simulink subsystem "Controls"  (R2024b)
settings: Solver=VariableStepAuto  StartTime=0.0  StopTime=10.0  RelTol=1e-3
undefined symbols (not defined in the file): D1, DiscIntNeverNeededParam, lag, Tctrl, test_alpha, Ts, Yg
libraries: powerlib_extras x74, simulink x10
(part 7 of 7)

== system Controls/Pole 2 Rectifier Control and Protection/Rectifier Controller/Voltage Regulator/Voltage Regulator/Kp Linearisation ==
  note: Kp Linearization
  Alpha_lin : Inport
  Kp : Inport  Port=2
  Inv : Inport  Port=3
  Min_lin : Inport  Port=4
  Max_lin : Inport  Port=5
  Constant3 : Constant  Value=On_lin
  Data Type Conversion : DataTypeConversion  OutDataTypeStr=boolean
  Logical Operator : Logic  Operator=NOT
  Logical Operator1 : Logic  Operator=NOT
  Math Function : Math  Operator=reciprocal  SignedPower=on
  Prod2 : Product  Inputs=3  InputSameDT=on  SaturateOnIntegerOverflow=on  OutDataTypeStr=Inherit: Same as first input
  S6 : Subsystem  mask(Limiter with External Limits){}
      mask Display: disp('      Limiter\n')
  Switch : Switch  Threshold=0.5
  Switch1 : Switch  Threshold=0.5
  Trigonometric Function : Trigonometry
  Trigonometric Function1 : Trigonometry
  k : Gain  Gain=pi/180  SaturateOnIntegerOverflow=on  OutDataTypeStr=Inherit: Same as input  ParamDataTypeStr=Inherit: Same as input
  k1 : Gain  Gain=pi/180  SaturateOnIntegerOverflow=on  OutDataTypeStr=Inherit: Same as input  ParamDataTypeStr=Inherit: Same as input
  Kp_lin : Outport  InitialOutput=0
  wires:
  Min_lin/1 -> S6/3(MIN), Switch/1
  Max_lin/1 -> S6/1(MAX), Switch/3
  Alpha_lin/1 -> S6/2(In)
  Math Function/1 -> Prod2/2
  Trigonometric Function1/1 -> Math Function/1
  k/1 -> Trigonometric Function1/1
  Kp/1 -> Prod2/3, Switch1/1
  Inv/1 -> Logical Operator/1
  Logical Operator/1 -> Switch/2
  Trigonometric Function/1 -> Prod2/1
  S6/1("  ") -> k/1
  k1/1 -> Trigonometric Function/1
  Switch/1 -> k1/1
  Switch1/1 -> Kp_lin/1
  Prod2/1 -> Switch1/3
  Logical Operator1/1 -> Switch1/2  "Off"
  Constant3/1 -> Data Type Conversion/1
  Data Type Conversion/1 -> Logical Operator1/1

== system Controls/Pole 2 Rectifier Control and Protection/Rectifier Controller/Voltage Regulator/Voltage Regulator/S16 ==
  note: INTEGRATOR with External limits & Reset & Hold
  note: Gain * dt
  Max : Inport
  Min : Inport  Port=2
  In : Inport  Port=3
  Reset : Inport  Port=4
  Hold : Inport  Port=5
  Reset Value : Inport  Port=6
  Gain1 : Gain  Gain=k*st  SaturateOnIntegerOverflow=on  OutDataTypeStr=Inherit: Same as input  ParamDataTypeStr=Inherit: Same as input
  IC = ic : UnitDelay  InitialCondition=ic  SampleTime=st  HasFrameUpgradeWarning=on
  Logical Operator4 : Logic  Operator=OR
  MinMax : MinMax  Inputs=2  InputSameDT=on  SaturateOnIntegerOverflow=on
  MinMax1 : MinMax  Function=max  Inputs=2  InputSameDT=on  SaturateOnIntegerOverflow=on
  S6 : Subsystem  mask(Limiter with External Limits){}
      mask Display: disp('      Limiter\n')
  Sum : Sum  InputSameDT=on  SaturateOnIntegerOverflow=on  OutDataTypeStr=Inherit: Same as first input
  Switch2 : Switch  Threshold=0.5
  Switch3 : Switch  Threshold=0.5
  Switch7 : Switch  Threshold=0.5
  Out : Outport  InitialOutput=0
  wires:
  Gain1/1 -> Sum/1
  In/1 -> Gain1/1
  Sum/1 -> S6/2(In)
  S6/1("  ") -> Out/1, IC = ic/1
  Hold/1 -> Logical Operator4/1
  Reset/1 -> Switch7/2, Logical Operator4/2
  Logical Operator4/1 -> Switch2/2, Switch3/2
  Switch2/1 -> MinMax/1
  Max/1 -> Switch2/3, MinMax/2
  Reset Value/1 -> Switch7/1
  MinMax/1 -> S6/1(MAX)
  MinMax1/1 -> S6/3(MIN)
  Switch3/1 -> MinMax1/1
  Min/1 -> Switch3/3, MinMax1/2
  IC = ic/1 -> Switch7/3
  Switch7/1 -> Switch2/1, Sum/2, Switch3/1

== system Controls/Pole 2 Rectifier Control and Protection/Rectifier Controller/Voltage Regulator/Voltage Regulator/S6 ==
  note: Limiter
      | with external
      | limits
  MAX : Inport
  In : Inport  Port=2
  MIN : Inport  Port=3
  MinMax : MinMax  Function=max  Inputs=2  InputSameDT=on  SaturateOnIntegerOverflow=on
  MinMax1 : MinMax  Inputs=2  InputSameDT=on  SaturateOnIntegerOverflow=on
  "  " : Outport  InitialOutput=0
  wires:
  In/1 -> MinMax1/2
  MinMax/1 -> "  "/1
  MIN/1 -> MinMax/1
  MAX/1 -> MinMax1/1
  MinMax1/1 -> MinMax/2

== system Controls/Pole 2 Rectifier Control and Protection/Rectifier Protections/DC Fault Protection (DCPROT)/Enabled Subsystem/Discrete Off Delay ==
  note: Discrete On/Off Delay
  note: Silvano Casoria
      | Power System Simulation Laboratory
      | IREQ, Hydro-Quebc
  IN : Inport
  Constant : Constant
  Constant1 : Constant  Value=delay - eps
  Constant2 : Constant  Value=type_delay
  Data Type Conversion1 : DataTypeConversion  OutDataTypeStr=boolean
  Logical Operator1 : Logic  Operator=OR
  Logical Operator2 : Logic  Operator=NOT  Inputs=1
  OFF Delay : Subsystem  TreatAsAtomicUnit=on
  ON Delay : Subsystem  TreatAsAtomicUnit=on
  Relational Operator1 : RelationalOperator  Operator===
  OUT : Outport  VectorParamsAs1DForOutWhenUnconnected=off
  wires:
  IN/1 -> Data Type Conversion1/1
  Constant1/1 -> OFF Delay/2(DELAY), ON Delay/2(DELAY)
  Logical Operator1/1 -> OUT/1
  ON Delay/1(OUT) -> Logical Operator1/1
  OFF Delay/1(OUT) -> Logical Operator1/2
  Logical Operator2/1 -> ?
  Constant2/1 -> Relational Operator1/1
  Relational Operator1/1 -> Logical Operator2/1, ON Delay/Enable
  Constant/1 -> Relational Operator1/2
  Data Type Conversion1/1 -> OFF Delay/1(IN), ON Delay/1(IN)

== system Controls/Pole 1 Inverter Control and Protection/Inverter Current //Voltage//Gamma Controller /Gamma Regulator/Gamma Regulator/Kp Linearisation/S6 ==
  note: Limiter
      | with external
      | limits
  MAX : Inport
  In : Inport  Port=2
  MIN : Inport  Port=3
  MinMax : MinMax  Function=max  Inputs=2  InputSameDT=on  SaturateOnIntegerOverflow=on
  MinMax1 : MinMax  Inputs=2  InputSameDT=on  SaturateOnIntegerOverflow=on
  "  " : Outport  InitialOutput=0
  wires:
  MinMax1/1 -> MinMax/2
  MAX/1 -> MinMax1/1
  MIN/1 -> MinMax/1
  MinMax/1 -> "  "/1
  In/1 -> MinMax1/2

== system Controls/Pole 1 Inverter Control and Protection/Inverter Current //Voltage//Gamma Controller /Gamma Regulator/Gamma Regulator/S16/S6 ==
  note: Silvano Casoria
      | Laboratoire simulation de reseaux, IREQ
  note: Limiter
      | with external
      | limits
  MAX : Inport
  In : Inport  Port=2
  MIN : Inport  Port=3
  MinMax : MinMax  Function=max  Inputs=2  InputSameDT=on  SaturateOnIntegerOverflow=on
  MinMax1 : MinMax  Inputs=2  InputSameDT=on  SaturateOnIntegerOverflow=on
  "  " : Outport  InitialOutput=0
  wires:
  In/1 -> MinMax1/2
  MinMax/1 -> "  "/1
  MIN/1 -> MinMax/1
  MAX/1 -> MinMax1/1
  MinMax1/1 -> MinMax/2

== system Controls/Pole 1 Inverter Control and Protection/Inverter Current //Voltage//Gamma Controller /Voltage Regulator/Voltage Regulator/Kp Linearisation/S6 ==
  note: Limiter
      | with external
      | limits
  MAX : Inport
  In : Inport  Port=2
  MIN : Inport  Port=3
  MinMax : MinMax  Function=max  Inputs=2  InputSameDT=on  SaturateOnIntegerOverflow=on
  MinMax1 : MinMax  Inputs=2  InputSameDT=on  SaturateOnIntegerOverflow=on
  "  " : Outport  InitialOutput=0
  wires:
  In/1 -> MinMax1/2
  MinMax/1 -> "  "/1
  MIN/1 -> MinMax/1
  MAX/1 -> MinMax1/1
  MinMax1/1 -> MinMax/2

== system Controls/Pole 1 Inverter Control and Protection/Inverter Current //Voltage//Gamma Controller /Voltage Regulator/Voltage Regulator/S16/S6 ==
  note: Limiter
      | with external
      | limits
  note: Silvano Casoria
      | Laboratoire simulation de reseaux, IREQ
  MAX : Inport
  In : Inport  Port=2
  MIN : Inport  Port=3
  MinMax : MinMax  Function=max  Inputs=2  InputSameDT=on  SaturateOnIntegerOverflow=on
  MinMax1 : MinMax  Inputs=2  InputSameDT=on  SaturateOnIntegerOverflow=on
  "  " : Outport  InitialOutput=0
  wires:
  MinMax1/1 -> MinMax/2
  MAX/1 -> MinMax1/1
  MIN/1 -> MinMax/1
  MinMax/1 -> "  "/1
  In/1 -> MinMax1/2

== system Controls/Pole 1 Rectifier Control and Protection/Rectifier Controller/Gamma Regulator/Gamma Regulator/Kp Linearisation/S6 ==
  note: Limiter
      | with external
      | limits
  MAX : Inport
  In : Inport  Port=2
  MIN : Inport  Port=3
  MinMax : MinMax  Function=max  Inputs=2  InputSameDT=on  SaturateOnIntegerOverflow=on
  MinMax1 : MinMax  Inputs=2  InputSameDT=on  SaturateOnIntegerOverflow=on
  "  " : Outport  InitialOutput=0
  wires:
  MinMax1/1 -> MinMax/2
  MAX/1 -> MinMax1/1
  MIN/1 -> MinMax/1
  MinMax/1 -> "  "/1
  In/1 -> MinMax1/2

== system Controls/Pole 1 Rectifier Control and Protection/Rectifier Controller/Gamma Regulator/Gamma Regulator/S16/S6 ==
  note: Silvano Casoria
      | Laboratoire simulation de reseaux, IREQ
  note: Limiter
      | with external
      | limits
  MAX : Inport
  In : Inport  Port=2
  MIN : Inport  Port=3
  MinMax : MinMax  Function=max  Inputs=2  InputSameDT=on  SaturateOnIntegerOverflow=on
  MinMax1 : MinMax  Inputs=2  InputSameDT=on  SaturateOnIntegerOverflow=on
  "  " : Outport  InitialOutput=0
  wires:
  In/1 -> MinMax1/2
  MinMax/1 -> "  "/1
  MIN/1 -> MinMax/1
  MAX/1 -> MinMax1/1
  MinMax1/1 -> MinMax/2

== system Controls/Pole 1 Rectifier Control and Protection/Rectifier Controller/Voltage Regulator/Voltage Regulator/Kp Linearisation/S6 ==
  note: Limiter
      | with external
      | limits
  MAX : Inport
  In : Inport  Port=2
  MIN : Inport  Port=3
  MinMax : MinMax  Function=max  Inputs=2  InputSameDT=on  SaturateOnIntegerOverflow=on
  MinMax1 : MinMax  Inputs=2  InputSameDT=on  SaturateOnIntegerOverflow=on
  "  " : Outport  InitialOutput=0
  wires:
  In/1 -> MinMax1/2
  MinMax/1 -> "  "/1
  MIN/1 -> MinMax/1
  MAX/1 -> MinMax1/1
  MinMax1/1 -> MinMax/2

== system Controls/Pole 1 Rectifier Control and Protection/Rectifier Controller/Voltage Regulator/Voltage Regulator/S16/S6 ==
  note: Limiter
      | with external
      | limits
  note: Silvano Casoria
      | Laboratoire simulation de reseaux, IREQ
  MAX : Inport
  In : Inport  Port=2
  MIN : Inport  Port=3
  MinMax : MinMax  Function=max  Inputs=2  InputSameDT=on  SaturateOnIntegerOverflow=on
  MinMax1 : MinMax  Inputs=2  InputSameDT=on  SaturateOnIntegerOverflow=on
  "  " : Outport  InitialOutput=0
  wires:
  MinMax1/1 -> MinMax/2
  MAX/1 -> MinMax1/1
  MIN/1 -> MinMax/1
  MinMax/1 -> "  "/1
  In/1 -> MinMax1/2

== system Controls/Pole 1 Rectifier Control and Protection/Rectifier Protections/DC Fault Protection (DCPROT)/Enabled Subsystem/Discrete Off Delay/OFF Delay ==
  IN : Inport
  DELAY : Inport  Port=2
  Enable : EnablePort  PropagateVarSize=During execution
  Constant2 : Constant  Value=-Ts
  Constant3 : Constant  Value=Ts
  Discrete Edge Detector : powerlib_extras/Discrete  Control Blocks/Discrete Edge Detector  model=Falling  ic=ic  Ts=Ts
  Logical Operator1 : Logic
  Logical Operator2 : Logic  Operator=NOT
  Logical Operator3 : Logic  Operator=NOT
  Relational Operator : RelationalOperator  OutDataTypeStr=boolean
  Sum1 : Sum  Inputs=+-  InputSameDT=on  SaturateOnIntegerOverflow=on  OutDataTypeStr=Inherit: Same as first input
  Switch : Switch  Threshold=0.5
  Unit Delay : UnitDelay  SampleTime=Ts  HasFrameUpgradeWarning=on
  OUT : Outport  VectorParamsAs1DForOutWhenUnconnected=off
  wires:
  Logical Operator3/1 -> OUT/1
  Logical Operator2/1 -> Logical Operator1/1
  Constant2/1 -> Relational Operator/1
  Discrete Edge Detector/1 -> Switch/2
  DELAY/1 -> Switch/1
  Logical Operator1/1 -> Logical Operator3/1
  IN/1 -> Logical Operator2/1, Discrete Edge Detector/1
  Relational Operator/1 -> Logical Operator1/2
  Constant3/1 -> Sum1/2
  Switch/1 -> Sum1/1
  Sum1/1 -> Unit Delay/1, Relational Operator/2
  Unit Delay/1 -> Switch/3

== system Controls/Pole 1 Rectifier Control and Protection/Rectifier Protections/DC Fault Protection (DCPROT)/Enabled Subsystem/Discrete Off Delay/ON Delay ==
  IN : Inport
  DELAY : Inport  Port=2
  Enable : EnablePort  PropagateVarSize=During execution
  Constant2 : Constant  Value=-Ts
  Constant3 : Constant  Value=Ts
  Discrete Edge Detector : powerlib_extras/Discrete  Control Blocks/Discrete Edge Detector  model=Rising  ic=ic  Ts=Ts
  Logical Operator1 : Logic
  Relational Operator : RelationalOperator  OutDataTypeStr=boolean
  Sum1 : Sum  Inputs=+-  InputSameDT=on  SaturateOnIntegerOverflow=on  OutDataTypeStr=Inherit: Same as first input
  Switch : Switch  Threshold=0.5
  Unit Delay : UnitDelay  SampleTime=Ts  HasFrameUpgradeWarning=on
  OUT : Outport  VectorParamsAs1DForOutWhenUnconnected=off
  wires:
  Constant2/1 -> Relational Operator/1
  Discrete Edge Detector/1 -> Switch/2
  DELAY/1 -> Switch/1
  Logical Operator1/1 -> OUT/1
  IN/1 -> Logical Operator1/1, Discrete Edge Detector/1
  Relational Operator/1 -> Logical Operator1/2
  Constant3/1 -> Sum1/2
  Switch/1 -> Sum1/1
  Sum1/1 -> Relational Operator/2, Unit Delay/1
  Unit Delay/1 -> Switch/3

== system Controls/Pole 2 Inverter Control and Protection/Inverter Current //Voltage//Gamma Controller /Gamma Regulator/Gamma Regulator/Kp Linearisation/S6 ==
  note: Limiter
      | with external
      | limits
  MAX : Inport
  In : Inport  Port=2
  MIN : Inport  Port=3
  MinMax : MinMax  Function=max  Inputs=2  InputSameDT=on  SaturateOnIntegerOverflow=on
  MinMax1 : MinMax  Inputs=2  InputSameDT=on  SaturateOnIntegerOverflow=on
  "  " : Outport  InitialOutput=0
  wires:
  MinMax1/1 -> MinMax/2
  MAX/1 -> MinMax1/1
  MIN/1 -> MinMax/1
  MinMax/1 -> "  "/1
  In/1 -> MinMax1/2

== system Controls/Pole 2 Inverter Control and Protection/Inverter Current //Voltage//Gamma Controller /Gamma Regulator/Gamma Regulator/S16/S6 ==
  note: Silvano Casoria
      | Laboratoire simulation de reseaux, IREQ
  note: Limiter
      | with external
      | limits
  MAX : Inport
  In : Inport  Port=2
  MIN : Inport  Port=3
  MinMax : MinMax  Function=max  Inputs=2  InputSameDT=on  SaturateOnIntegerOverflow=on
  MinMax1 : MinMax  Inputs=2  InputSameDT=on  SaturateOnIntegerOverflow=on
  "  " : Outport  InitialOutput=0
  wires:
  In/1 -> MinMax1/2
  MinMax/1 -> "  "/1
  MIN/1 -> MinMax/1
  MAX/1 -> MinMax1/1
  MinMax1/1 -> MinMax/2

== system Controls/Pole 2 Inverter Control and Protection/Inverter Current //Voltage//Gamma Controller /Voltage Regulator/Voltage Regulator/Kp Linearisation/S6 ==
  note: Limiter
      | with external
      | limits
  MAX : Inport
  In : Inport  Port=2
  MIN : Inport  Port=3
  MinMax : MinMax  Function=max  Inputs=2  InputSameDT=on  SaturateOnIntegerOverflow=on
  MinMax1 : MinMax  Inputs=2  InputSameDT=on  SaturateOnIntegerOverflow=on
  "  " : Outport  InitialOutput=0
  wires:
  In/1 -> MinMax1/2
  MinMax/1 -> "  "/1
  MIN/1 -> MinMax/1
  MAX/1 -> MinMax1/1
  MinMax1/1 -> MinMax/2

== system Controls/Pole 2 Inverter Control and Protection/Inverter Current //Voltage//Gamma Controller /Voltage Regulator/Voltage Regulator/S16/S6 ==
  note: Limiter
      | with external
      | limits
  note: Silvano Casoria
      | Laboratoire simulation de reseaux, IREQ
  MAX : Inport
  In : Inport  Port=2
  MIN : Inport  Port=3
  MinMax : MinMax  Function=max  Inputs=2  InputSameDT=on  SaturateOnIntegerOverflow=on
  MinMax1 : MinMax  Inputs=2  InputSameDT=on  SaturateOnIntegerOverflow=on
  "  " : Outport  InitialOutput=0
  wires:
  MinMax1/1 -> MinMax/2
  MAX/1 -> MinMax1/1
  MIN/1 -> MinMax/1
  MinMax/1 -> "  "/1
  In/1 -> MinMax1/2

== system Controls/Pole 2 Rectifier Control and Protection/Rectifier Controller/Gamma Regulator/Gamma Regulator/Kp Linearisation/S6 ==
  note: Limiter
      | with external
      | limits
  MAX : Inport
  In : Inport  Port=2
  MIN : Inport  Port=3
  MinMax : MinMax  Function=max  Inputs=2  InputSameDT=on  SaturateOnIntegerOverflow=on
  MinMax1 : MinMax  Inputs=2  InputSameDT=on  SaturateOnIntegerOverflow=on
  "  " : Outport  InitialOutput=0
  wires:
  MinMax1/1 -> MinMax/2
  MAX/1 -> MinMax1/1
  MIN/1 -> MinMax/1
  MinMax/1 -> "  "/1
  In/1 -> MinMax1/2

== system Controls/Pole 2 Rectifier Control and Protection/Rectifier Controller/Gamma Regulator/Gamma Regulator/S16/S6 ==
  note: Silvano Casoria
      | Laboratoire simulation de reseaux, IREQ
  note: Limiter
      | with external
      | limits
  MAX : Inport
  In : Inport  Port=2
  MIN : Inport  Port=3
  MinMax : MinMax  Function=max  Inputs=2  InputSameDT=on  SaturateOnIntegerOverflow=on
  MinMax1 : MinMax  Inputs=2  InputSameDT=on  SaturateOnIntegerOverflow=on
  "  " : Outport  InitialOutput=0
  wires:
  In/1 -> MinMax1/2
  MinMax/1 -> "  "/1
  MIN/1 -> MinMax/1
  MAX/1 -> MinMax1/1
  MinMax1/1 -> MinMax/2

== system Controls/Pole 2 Rectifier Control and Protection/Rectifier Controller/Voltage Regulator/Voltage Regulator/Kp Linearisation/S6 ==
  note: Limiter
      | with external
      | limits
  MAX : Inport
  In : Inport  Port=2
  MIN : Inport  Port=3
  MinMax : MinMax  Function=max  Inputs=2  InputSameDT=on  SaturateOnIntegerOverflow=on
  MinMax1 : MinMax  Inputs=2  InputSameDT=on  SaturateOnIntegerOverflow=on
  "  " : Outport  InitialOutput=0
  wires:
  In/1 -> MinMax1/2
  MinMax/1 -> "  "/1
  MIN/1 -> MinMax/1
  MAX/1 -> MinMax1/1
  MinMax1/1 -> MinMax/2

== system Controls/Pole 2 Rectifier Control and Protection/Rectifier Controller/Voltage Regulator/Voltage Regulator/S16/S6 ==
  note: Limiter
      | with external
      | limits
  note: Silvano Casoria
      | Laboratoire simulation de reseaux, IREQ
  MAX : Inport
  In : Inport  Port=2
  MIN : Inport  Port=3
  MinMax : MinMax  Function=max  Inputs=2  InputSameDT=on  SaturateOnIntegerOverflow=on
  MinMax1 : MinMax  Inputs=2  InputSameDT=on  SaturateOnIntegerOverflow=on
  "  " : Outport  InitialOutput=0
  wires:
  MinMax1/1 -> MinMax/2
  MAX/1 -> MinMax1/1
  MIN/1 -> MinMax/1
  MinMax/1 -> "  "/1
  In/1 -> MinMax1/2

== system Controls/Pole 2 Rectifier Control and Protection/Rectifier Protections/DC Fault Protection (DCPROT)/Enabled Subsystem/Discrete Off Delay/OFF Delay ==
  IN : Inport
  DELAY : Inport  Port=2
  Constant2 : Constant  Value=-Ts
  Constant3 : Constant  Value=Ts
  Discrete Edge Detector : powerlib_extras/Discrete  Control Blocks/Discrete Edge Detector  model=Falling  ic=ic  Ts=Ts
  Logical Operator1 : Logic
  Logical Operator2 : Logic  Operator=NOT
  Logical Operator3 : Logic  Operator=NOT
  Relational Operator : RelationalOperator  OutDataTypeStr=boolean
  Sum1 : Sum  Inputs=+-  InputSameDT=on  SaturateOnIntegerOverflow=on  OutDataTypeStr=Inherit: Same as first input
  Switch : Switch  Threshold=0.5
  Unit Delay : UnitDelay  SampleTime=Ts  HasFrameUpgradeWarning=on
  OUT : Outport  VectorParamsAs1DForOutWhenUnconnected=off
  wires:
  Logical Operator3/1 -> OUT/1
  Logical Operator2/1 -> Logical Operator1/1
  Constant2/1 -> Relational Operator/1
  Discrete Edge Detector/1 -> Switch/2
  DELAY/1 -> Switch/1
  Logical Operator1/1 -> Logical Operator3/1
  IN/1 -> Logical Operator2/1, Discrete Edge Detector/1
  Relational Operator/1 -> Logical Operator1/2
  Constant3/1 -> Sum1/2
  Switch/1 -> Sum1/1
  Sum1/1 -> Unit Delay/1, Relational Operator/2
  Unit Delay/1 -> Switch/3

== system Controls/Pole 2 Rectifier Control and Protection/Rectifier Protections/DC Fault Protection (DCPROT)/Enabled Subsystem/Discrete Off Delay/ON Delay ==
  IN : Inport
  DELAY : Inport  Port=2
  Enable : EnablePort  PropagateVarSize=During execution
  Constant2 : Constant  Value=-Ts
  Constant3 : Constant  Value=Ts
  Discrete Edge Detector : powerlib_extras/Discrete  Control Blocks/Discrete Edge Detector  model=Rising  ic=ic  Ts=Ts
  Logical Operator1 : Logic
  Relational Operator : RelationalOperator  OutDataTypeStr=boolean
  Sum1 : Sum  Inputs=+-  InputSameDT=on  SaturateOnIntegerOverflow=on  OutDataTypeStr=Inherit: Same as first input
  Switch : Switch  Threshold=0.5
  Unit Delay : UnitDelay  SampleTime=Ts  HasFrameUpgradeWarning=on
  OUT : Outport  VectorParamsAs1DForOutWhenUnconnected=off
  wires:
  Constant2/1 -> Relational Operator/1
  Discrete Edge Detector/1 -> Switch/2
  DELAY/1 -> Switch/1
  Logical Operator1/1 -> OUT/1
  IN/1 -> Logical Operator1/1, Discrete Edge Detector/1
  Relational Operator/1 -> Logical Operator1/2
  Constant3/1 -> Sum1/2
  Switch/1 -> Sum1/1
  Sum1/1 -> Relational Operator/2, Unit Delay/1
  Unit Delay/1 -> Switch/3
